simulink library "LoadLib"  (R2021b)
settings: Solver=VariableStepAuto  StartTime=0.0  StopTime=10.0  RelTol=1e-3
values from neighbouring files (symbols this model uses):
  loadcoeff = 1.0    (= 1)    [init_IEEE34nodetestfeeder.m]
  VsubL = 24.9e3    (= 24900)    [init_IEEE34nodetestfeeder.m]
undefined symbols (not defined in the file or in its folder): DiscIntNeverNeededParam, SinglePhase_PQLoad, SinglePhase_PQLoadwithFeedForwardwoFilter_woFreqDependency
libraries: simulink_extras x2, spsDynamicLoadModel x2, spsControlledCurrentSourceLib x1, spsSeriesRLCBranchLib x1, simulink x1, spsVoltageMeasurementLib x1
settings Model: Creator=gl8300  LastModifiedBy=gl8300

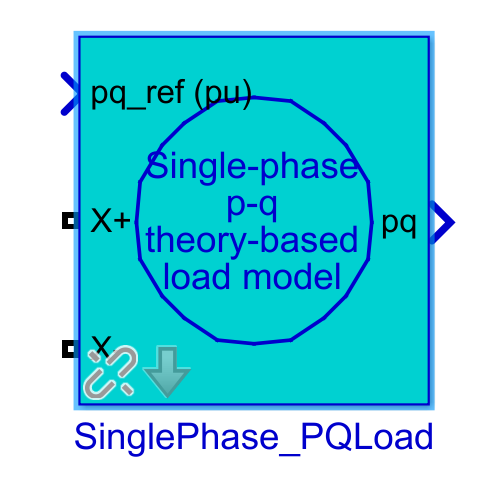
[thumbnail: Simulink's stored preview of the top-level diagram]
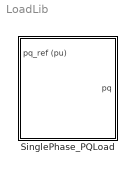
== system LoadLib ==
  SinglePhase_PQLoad : Subsystem  AncestorBlock=SinglePhase_PQLoad/SinglePhase_PQLoadwithFeedForwardwoFilter_woFreqDependency  mask(Single-phase dynamic load){fnom=60, Vbase=VsubL/sqrt(3), V0=1, S0=[4*1000*loadcoeff 2*1000*loadcoeff]/50e3, PQext=off, Kpi=[0.01 690], BasePower=50e3, n=[2 2], T=[0 0 0 0], Vmin=0.7, Freq_dep=on, FKpq=[0 0], Ts=50e-6}
      mask prompts: fnom "Nominal frequency [Hz]:"; Vbase "Nominal voltage [Vn(Vrms)]"; V0 "Initial positive-sequence voltage Vo [Mag(pu)]"; S0 "Active and reactive power at initial voltage [Po(pu) Qo(pu)]:"; PQext "External control of PQ"; Kpi "Active and Reactive power control parameters [Kp Ki]"; BasePower "Base Power (VA)"; n "[np, nq]:"; T "Time constants [Tp1 Tp2 Tq1 Tq2]  (s):"; Vmin "Minimum voltage Vmin (pu)"; Freq_dep "Frequency dependency"; FKpq "Frequency Dependency Gains [Kpf Kqf]"; Ts "Sample time (s)"
      mask help: Single-phase dynamic load based on p-q theory
      mask init:
      | wn=2*pi*fnom;
      | T1=1/wn;
      | Tp1=T(1);
      | Tp2=T(2);
      | Tq1=T(3);
      | Tq2=T(4);
      | P0=S0(1);
      | Q0=S0(2);
      | np=n(1);
      | nq=n(2);
      | Kpf=FKpq(1);
      | Kqf=FKpq(2);
      | K_SOGI = sqrt(2);
      | T=46;
      mask Callback PQext:
      | PQext = get_param(gcb,'PQext');
      | if strcmp(PQext,'on')
      |     set_param(gcb,'MaskEnables',{'on','on','off','off','on','on','on','off','off','off','off','off','on'});
      | else
      |     set_param(gcb,'MaskEnables',{'on','on','on','on','on','on','on','on','on','on','on','on','on'});
      | end
      mask Display:
      | %plot(-45,-45,45,45,[0,9,18,24,29,30,29,24,18,9,0,-9,-18,-24,-29,-30,-29,-24,-18,-9,0]*.9,[30,29,24,18,9,0,-9,-18,-24,-29,-30,-29,-24,-18,-9,0,9,18,24,29,30]*.9)
      | %plot([0,0,10,0,-10,0]*1.1,[15,-5,-5,-15,-5,-5]*1.1)
      | plot(-40,-40,40,40,[0,9,18,24,29,30,29,24,18,9,0,-9,-18,-24,-29,-30,-29,-24,-18,-9,0]*.9,[30,29,24,18,9,0,-9,-18,-24,-29,-30,-29,-24,-18,-9,0,9,18,24,29,30]*.9)
      | disp('Single-phase\np-q\ntheory-based\nload model')

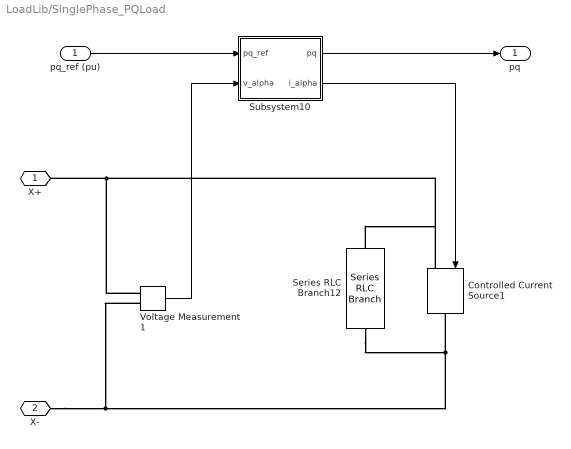
== system LoadLib/SinglePhase_PQLoad ==
  pq_ref (pu) : Inport
  Controlled Current Source1 : spsControlledCurrentSourceLib/Controlled Current Source  Initialize=on  Source_Type=AC  Amplitude=0  Phase=0  Frequency=0  Measurements=None
  Series RLC Branch12 : spsSeriesRLCBranchLib/Series RLC Branch  LConnTagsString=__new0  RConnTagsString=__new0  BranchType=R  Resistance=1e8  Inductance=1e-3  SetiL0=off  InitialCurrent=0  Capacitance=1e-6  Setx0=off  InitialVoltage=0  Measurements=None
  Subsystem10 : Subsystem
  Voltage Measurement1 : spsVoltageMeasurementLib/Voltage Measurement  PhasorSimulation=off  OutputType=Complex  PSBequivalent=0
  X+ : PMIOPort  Side=Left
  X- : PMIOPort  Port=2  Side=Left
  pq : Outport
  wires:
  Voltage Measurement1/1 -> Subsystem10/2(v_alpha)
  pq_ref (pu)/1 -> Subsystem10/1(pq_ref)
  Subsystem10/2(i_alpha) -> Controlled Current Source1/1
  Subsystem10/1(pq) -> pq/1
  connections:
  Voltage Measurement1/LConn2 -- X-/RConn1 -- Controlled Current Source1/RConn1 -- Series RLC Branch12/RConn1
  Voltage Measurement1/LConn1 -- Series RLC Branch12/LConn1 -- Controlled Current Source1/LConn1 -- X+/RConn1

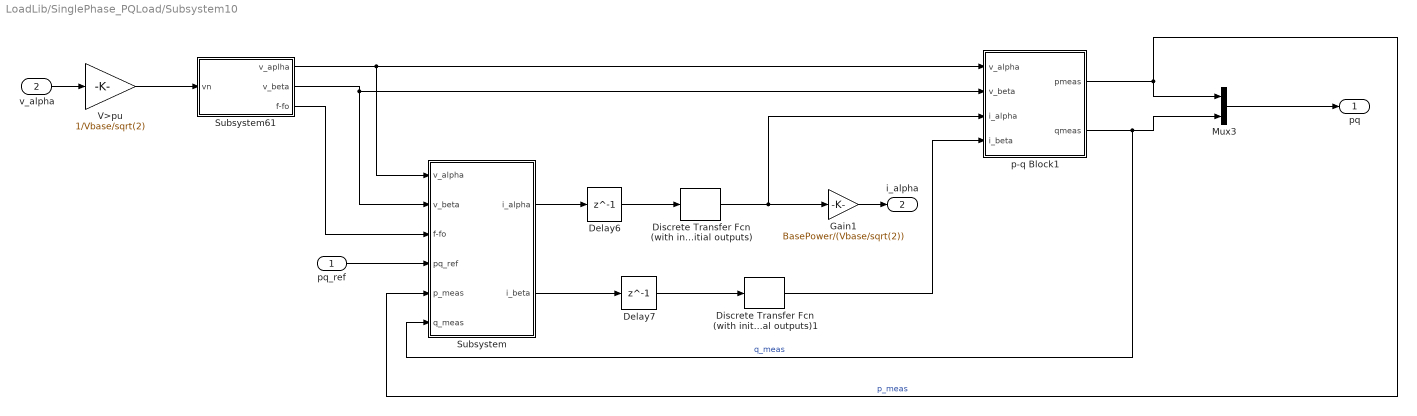
== system LoadLib/SinglePhase_PQLoad/Subsystem10 ==
  pq_ref : Inport
  v_alpha : Inport  Port=2
  Delay6 : Delay  DelayLength=1  InitialCondition=0
  Delay7 : Delay  DelayLength=1  InitialCondition=0
  Discrete Transfer Fcn (with initial outputs) : simulink_extras/Additional Discrete/Discrete Transfer Fcn (with initial outputs)  N=[0.00933705475365587 0.00933705475365587]  D=[1 -0.981325890492688]  U0=0.01  Y0=0.01  TS=Ts
      settings: SourceProductBaseCode=SL
  Discrete Transfer Fcn (with initial outputs)1 : simulink_extras/Additional Discrete/Discrete Transfer Fcn (with initial outputs)  N=[0.00933705475365587 0.00933705475365587]  D=[1 -0.981325890492688]  U0=0.01  Y0=0.01  TS=Ts
      settings: SourceProductBaseCode=SL
  Gain1 : Gain  Gain=BasePower/(Vbase/sqrt(2))
  Mux3 : Mux  Inputs=2
  Subsystem : Subsystem
  Subsystem61 : Subsystem
  V>pu : Gain  Gain=1/Vbase/sqrt(2)
  p-q Block1 : MATLAB Function  TreatAsAtomicUnit=on
  pq : Outport
  i_alpha : Outport  Port=2
  wires:
  V>pu/1 -> Subsystem61/1(vn)
  Subsystem61/2(v_beta) -> Subsystem/2(v_beta), p-q Block1/2(v_beta)
  Subsystem/2(i_beta) -> Delay7/1
  p-q Block1/2(qmeas) -> Subsystem/6(q_meas), Mux3/2  "q_meas"
  Subsystem/1(i_alpha) -> Delay6/1
  Mux3/1 -> pq/1
  pq_ref/1 -> Subsystem/4(pq_ref)
  v_alpha/1 -> V>pu/1
  p-q Block1/1(pmeas) -> Subsystem/5(p_meas), Mux3/1  "p_meas"
  Subsystem61/3(f-fo) -> Subsystem/3(f-fo)
  Delay6/1 -> Discrete Transfer Fcn (with initial outputs)/1
  Delay7/1 -> Discrete Transfer Fcn (with initial outputs)1/1
  Gain1/1 -> i_alpha/1
  Discrete Transfer Fcn (with initial outputs)/1 -> Gain1/1, p-q Block1/3(i_alpha)
  Discrete Transfer Fcn (with initial outputs)1/1 -> p-q Block1/4(i_beta)
  Subsystem61/1(v_aplha) -> p-q Block1/1(v_alpha), Subsystem/1(v_alpha)

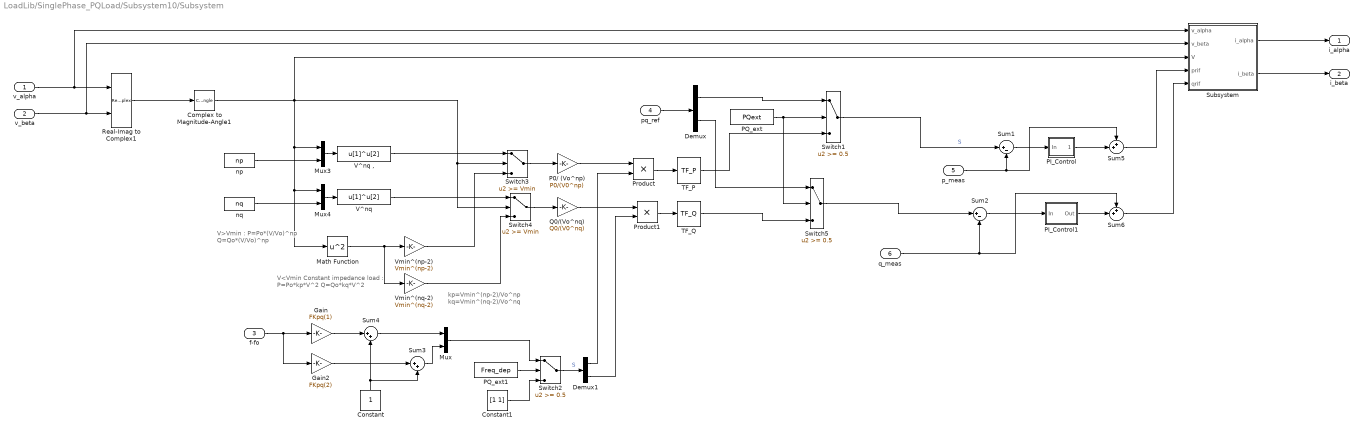
== system LoadLib/SinglePhase_PQLoad/Subsystem10/Subsystem ==
  note: V>Vmin :
      |
      |    P=Po*(V/Vo)^np
      |    Q=Qo*(V/Vo)^np
  note: kp=Vmin^(np-2)/Vo^np
      | kq=Vmin^(nq-2)/Vo^nq
  note: V<Vmin
      | Constant impedance load :
      |  P=Po*kp*V^2
      | Q=Qo*kq*V^2
  v_alpha : Inport
  v_beta : Inport  Port=2
  f-fo : Inport  Port=3
  pq_ref : Inport  Port=4
  p_meas : Inport  Port=5
  q_meas : Inport  Port=6
  Complex to Magnitude-Angle1 : ComplexToMagnitudeAngle  Output=Magnitude
  Constant : Constant
  Constant1 : Constant  Value=[1 1]
  Demux : Demux  Outputs=2
  Demux1 : Demux  Outputs=2
  Gain : Gain  Gain=FKpq(1)
  Gain2 : Gain  Gain=FKpq(2)
  Math Function : Math  Operator=square  SignedPower=on  SaturateOnIntegerOverflow=on
  Mux : Mux  Inputs=2
  Mux3 : Mux  Inputs=2
  Mux4 : Mux  Inputs=2
  P0/ (Vo^np) : Gain  Gain=P0/(V0^np)  SaturateOnIntegerOverflow=on  OutDataTypeStr=Inherit: Same as input  ParamDataTypeStr=Inherit: Same as input
  PI_Control : Subsystem
  PI_Control1 : Subsystem
  PQ_ext : Constant  Value=PQext
  PQ_ext1 : Constant  Value=Freq_dep
  Product : Product
  Product1 : Product
  Q0/(Vo^nq) : Gain  Gain=Q0/(V0^nq)  SaturateOnIntegerOverflow=on  OutDataTypeStr=Inherit: Same as input  ParamDataTypeStr=Inherit: Same as input
  Real-Imag to Complex1 : RealImagToComplex
  Subsystem : Subsystem
  Sum1 : Sum  Inputs=|+-
  Sum2 : Sum  Inputs=|+-
  Sum3 : Sum  Inputs=|++
  Sum4 : Sum  Inputs=|++
  Sum5 : Sum  Inputs=++|
  Sum6 : Sum  Inputs=++|
  Switch1 : Switch  Threshold=0.5  InputSameDT=on
  Switch2 : Switch  Threshold=0.5  InputSameDT=on
  Switch3 : Switch  Threshold=Vmin  InputSameDT=on
  Switch4 : Switch  Threshold=Vmin  InputSameDT=on
  Switch5 : Switch  Threshold=0.5  InputSameDT=on
  TF_P : spsDynamicLoadModel/Discrete/Positive Sequence  current/TF_P  T1=Tp1  T2=Tp2  V_Init=P0  Ts=Ts
      settings: SourceProductBaseCode=PS
  TF_Q : spsDynamicLoadModel/Discrete/Positive Sequence  current/TF_Q  T1=Tq1  T2=Tq2  V_Init=Q0  Ts=Ts
      settings: SourceProductBaseCode=PS
  V^nq : Fcn  Expr=u[1]^u[2]
  V^nq , : Fcn  Expr=u[1]^u[2]
  Vmin^(np-2) : Gain  Gain=Vmin^(np-2)  SaturateOnIntegerOverflow=on  OutDataTypeStr=Inherit: Same as input  ParamDataTypeStr=Inherit: Same as input
  Vmin^(nq-2) : Gain  Gain=Vmin^(nq-2)  SaturateOnIntegerOverflow=on  OutDataTypeStr=Inherit: Same as input  ParamDataTypeStr=Inherit: Same as input
  np : Constant  Value=np
  nq : Constant  Value=nq
  i_alpha : Outport
  i_beta : Outport  Port=2
  wires:
  pq_ref/1 -> Demux/1
  Demux/2 -> Switch5/1
  q_meas/1 -> Sum6/1, Sum2/2
  p_meas/1 -> Sum5/1, Sum1/2
  Demux/1 -> Switch1/1
  TF_Q/1 -> Switch5/3
  Sum1/1 -> PI_Control/1(In)
  Sum2/1 -> PI_Control1/1(In)
  Switch4/1 -> Q0/(Vo^nq)/1
  nq/1 -> Mux4/2
  Switch3/1 -> P0/ (Vo^np)/1
  v_beta/1 -> Real-Imag to Complex1/2, Subsystem/2(v_beta)
  Switch1/1 -> Sum1/1  "S"
  Real-Imag to Complex1/1 -> Complex to Magnitude-Angle1/1
  Vmin^(nq-2)/1 -> Switch4/3
  v_alpha/1 -> Subsystem/1(v_alpha), Real-Imag to Complex1/1
  V^nq/1 -> Switch4/1
  np/1 -> Mux3/2
  Vmin^(np-2)/1 -> Switch3/3
  Math Function/1 -> Vmin^(np-2)/1, Vmin^(nq-2)/1
  Mux4/1 -> V^nq/1
  Mux3/1 -> V^nq ,/1
  PQ_ext/1 -> Switch5/2, Switch1/2
  TF_P/1 -> Switch1/3
  V^nq ,/1 -> Switch3/1
  Switch5/1 -> Sum2/1
  Subsystem/2(i_beta) -> i_beta/1
  Subsystem/1(i_alpha) -> i_alpha/1
  Constant/1 -> Sum3/2, Sum4/2
  Sum3/1 -> Mux/2
  Switch2/1 -> Demux1/1  "S"
  PQ_ext1/1 -> Switch2/2
  f-fo/1 -> Gain2/1, Gain/1
  Sum4/1 -> Mux/1
  Demux1/1 -> Product/2
  Gain/1 -> Sum4/1
  Gain2/1 -> Sum3/1
  Demux1/2 -> Product1/2
  P0/ (Vo^np)/1 -> Product/1
  Product/1 -> TF_P/1
  Q0/(Vo^nq)/1 -> Product1/1
  Product1/1 -> TF_Q/1
  Sum5/1 -> Subsystem/4(prif)
  Sum6/1 -> Subsystem/5(qrif)
  PI_Control1/1(Out) -> Sum6/2
  PI_Control/1(Out) -> Sum5/2
  Complex to Magnitude-Angle1/1 -> Mux3/1, Mux4/1, Math Function/1, Subsystem/3(V), Switch4/2, Switch3/2
  Constant1/1 -> Switch2/3
  Mux/1 -> Switch2/1

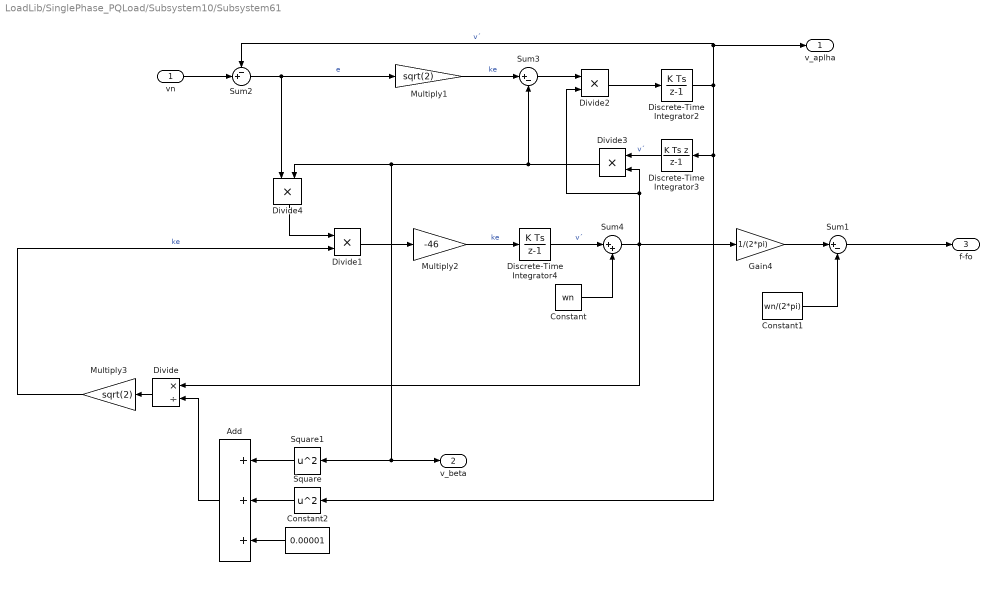
== system LoadLib/SinglePhase_PQLoad/Subsystem10/Subsystem61 ==
  vn : Inport
  Add : Sum  Inputs=+++
  Constant : Constant  Value=wn
  Constant1 : Constant  Value=wn/(2*pi)
  Constant2 : Constant  Value=0.00001
  Discrete-Time Integrator2 : DiscreteIntegrator  SampleTime=-1  ICPrevOutput=DiscIntNeverNeededParam  ICPrevScaledInput=DiscIntNeverNeededParam
  Discrete-Time Integrator3 : DiscreteIntegrator  IntegratorMethod=Integration: Backward Euler  SampleTime=-1  ICPrevOutput=DiscIntNeverNeededParam  ICPrevScaledInput=DiscIntNeverNeededParam
  Discrete-Time Integrator4 : DiscreteIntegrator  SampleTime=-1  ICPrevOutput=DiscIntNeverNeededParam  ICPrevScaledInput=DiscIntNeverNeededParam
  Divide : Product  Inputs=*/
  Divide{1..4} (4 alike) : Product  Inputs=**
  Gain4 : Gain  Gain=1/(2*pi)
  Multiply1 : Gain  Gain=sqrt(2)
  Multiply2 : Gain  Gain=-46
  Multiply3 : Gain  Gain=sqrt(2)
  Square : Math  Operator=square  SaturateOnIntegerOverflow=on
  Square1 : Math  Operator=square  SaturateOnIntegerOverflow=on
  Sum1 : Sum  Inputs=|+-
  Sum2 : Sum  Inputs=-+|
  Sum3 : Sum  Inputs=|+-
  Sum4 : Sum  Inputs=|++
  v_aplha : Outport
  v_beta : Outport  Port=2
  f-fo : Outport  Port=3
  wires:
  Divide3/1 -> Divide4/2, Square1/1, v_beta/1, Sum3/2
  vn/1 -> Sum2/2
  Divide2/1 -> Discrete-Time Integrator2/1
  Discrete-Time Integrator2/1 -> Square/1, Discrete-Time Integrator3/1, v_aplha/1, Sum2/1  "v´"
  Discrete-Time Integrator4/1 -> Sum4/1  "v´"
  Sum2/1 -> Divide4/1, Multiply1/1  "e"
  Discrete-Time Integrator3/1 -> Divide3/1  "v´"
  Constant/1 -> Sum4/2
  Multiply2/1 -> Discrete-Time Integrator4/1  "ke"
  Multiply1/1 -> Sum3/1  "ke"
  Sum3/1 -> Divide2/1
  Square1/1 -> Add/1
  Square/1 -> Add/2
  Add/1 -> Divide/2
  Divide/1 -> Multiply3/1
  Divide1/1 -> Multiply2/1
  Divide4/1 -> Divide1/1
  Multiply3/1 -> Divide1/2  "ke"
  Constant2/1 -> Add/3
  Sum1/1 -> f-fo/1
  Constant1/1 -> Sum1/2
  Sum4/1 -> Gain4/1, Divide/1, Divide2/2, Divide3/2
  Gain4/1 -> Sum1/1

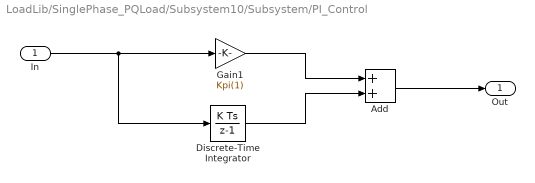
== system LoadLib/SinglePhase_PQLoad/Subsystem10/Subsystem/PI_Control ==
  In : Inport
  Add : Sum
  Discrete-Time Integrator : DiscreteIntegrator  gainval=Kpi(2)  SampleTime=-1  ICPrevOutput=DiscIntNeverNeededParam  ICPrevScaledInput=DiscIntNeverNeededParam
  Gain1 : Gain  Gain=Kpi(1)
  Out : Outport
  wires:
  In/1 -> Discrete-Time Integrator/1, Gain1/1
  Gain1/1 -> Add/1
  Add/1 -> Out/1
  Discrete-Time Integrator/1 -> Add/2

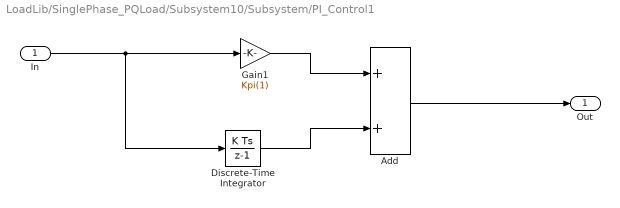
== system LoadLib/SinglePhase_PQLoad/Subsystem10/Subsystem/PI_Control1 ==
  In : Inport
  Add : Sum
  Discrete-Time Integrator : DiscreteIntegrator  gainval=Kpi(2)  SampleTime=-1  ICPrevOutput=DiscIntNeverNeededParam  ICPrevScaledInput=DiscIntNeverNeededParam
  Gain1 : Gain  Gain=Kpi(1)
  Out : Outport
  wires:
  In/1 -> Discrete-Time Integrator/1, Gain1/1
  Gain1/1 -> Add/1
  Discrete-Time Integrator/1 -> Add/2
  Add/1 -> Out/1

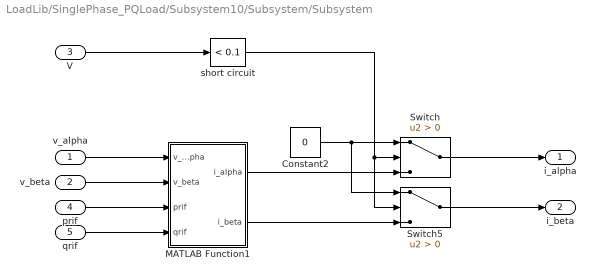
== system LoadLib/SinglePhase_PQLoad/Subsystem10/Subsystem/Subsystem ==
  v_alpha : Inport
  v_beta : Inport  Port=2
  V : Inport  Port=3
  prif : Inport  Port=4
  qrif : Inport  Port=5
  Constant2 : Constant  Value=0
  MATLAB Function1 : MATLAB Function  TreatAsAtomicUnit=on
  Switch : Switch  Criteria=u2 > Threshold
  Switch5 : Switch  Criteria=u2 > Threshold
  short circuit : simulink/Logic and Bit Operations/Compare To Constant  relop=<  const=0.1  OutDataTypeStr=boolean
  i_alpha : Outport
  i_beta : Outport  Port=2
  wires:
  MATLAB Function1/2(i_beta) -> Switch5/3
  V/1 -> short circuit/1
  v_alpha/1 -> MATLAB Function1/1(v_alpha)
  qrif/1 -> MATLAB Function1/4(qrif)
  Constant2/1 -> Switch/1, Switch5/1
  MATLAB Function1/1(i_alpha) -> Switch/3
  prif/1 -> MATLAB Function1/3(prif)
  v_beta/1 -> MATLAB Function1/2(v_beta)
  Switch/1 -> i_alpha/1
  Switch5/1 -> i_beta/1
  short circuit/1 -> Switch5/2, Switch/2

== matlab function LoadLib/SinglePhase_PQLoad/Subsystem10/Subsystem/Subsystem/MATLAB Function1 ==
  data: v_alpha input; i_alpha output; v_beta input; prif input; qrif input; i_beta output

function [i_alpha,i_beta]= fcn(v_alpha,v_beta,prif,qrif)
i_alpha=(v_alpha.*prif+v_beta.*qrif)/(v_alpha.^2+v_beta.^2);
i_beta=(v_beta.*prif-v_alpha.*qrif)/(v_alpha.^2+v_beta.^2);

== matlab function LoadLib/SinglePhase_PQLoad/Subsystem10/p-q Block1 ==
  data: v_alpha input; pmeas output; v_beta input; i_alpha input; i_beta input; qmeas output
function [pmeas,qmeas]= fcn(v_alpha,v_beta,i_alpha,i_beta)

pmeas=v_alpha.*i_alpha+v_beta.*i_beta;
qmeas=v_beta.*i_alpha-v_alpha.*i_beta;
